simulink model "3_Pose_integration_R_L"  (R2020b)
settings: Solver=FixedStepDiscrete  StartTime=0.0  StopTime=60  FixedStep=0.02  RelTol=1e-3  EnableMultiTasking=on
InitFcn:
  | load('Encoder_Data.mat')
StopFcn:
  | I = imread('Enviroment.png');
  | x = [0 35.9];
  | y=[23.31 0];
  | image(I,'XData',x,'YData',y);
  | axis xy;
  | hold on
  | plot (X.Data, Y.Data,'b');
  | plot (X1.Data, Y1.Data,'r');
undefined symbols (not defined in the file or in its folder): DiscIntNeverNeededParam, Ts
libraries: simulink x3
settings Model: Creator=antonio  LastModifiedBy=antonio
settings DataIOCC: LimitDataPoints=on  SaveFormat=Array  ReturnWorkspaceOutputs=off
settings OptimizationCC: LifeSpan=inf
settings DebuggingCC: UnderspecifiedInitializationDetection=Classic  MergeDetectMultiDrivingBlocksExec=none  SolverPrmCheckMsg=warning  StateNameClashWarn=warning  SFUnexpectedBacktrackingDiag=warning  SFNoUnconditionalDefaultTransitionDiag=warning  SFExecutionAtInitializationDiag=none  ArithmeticOperatorsInVariantConditions=warning
settings HardwareCC: ProdBitPerPointer=32  ProdBitPerSizeT=32  ProdBitPerPtrDiffT=32  ProdLargestAtomicFloat=None  ProdIntDivRoundTo=Undefined  ProdEndianess=Unspecified  ProdWordSize=32  ProdHWDeviceType=32-bit Generic
settings ModelReferenceCC: PropagateSignalLabelsOutOfModel=off
settings SFSimCC: SimUseLocalCustomCode=off  CustomCodeUndefinedFunction=UseInterfaceOnly
settings RTWCC: RTWUseLocalCustomCode=off
settings CodeAppCC: StateflowObjectComments=on
settings GRTTargetCC: TargetLangStandard=C89/C90 (ANSI)
settings ConfigComp: CovMetricSettings=dw  CovSaveCumulativeToWorkspaceVar=on  CovSaveSingleToWorkspaceVar=on  CovExternalEMLEnable=off

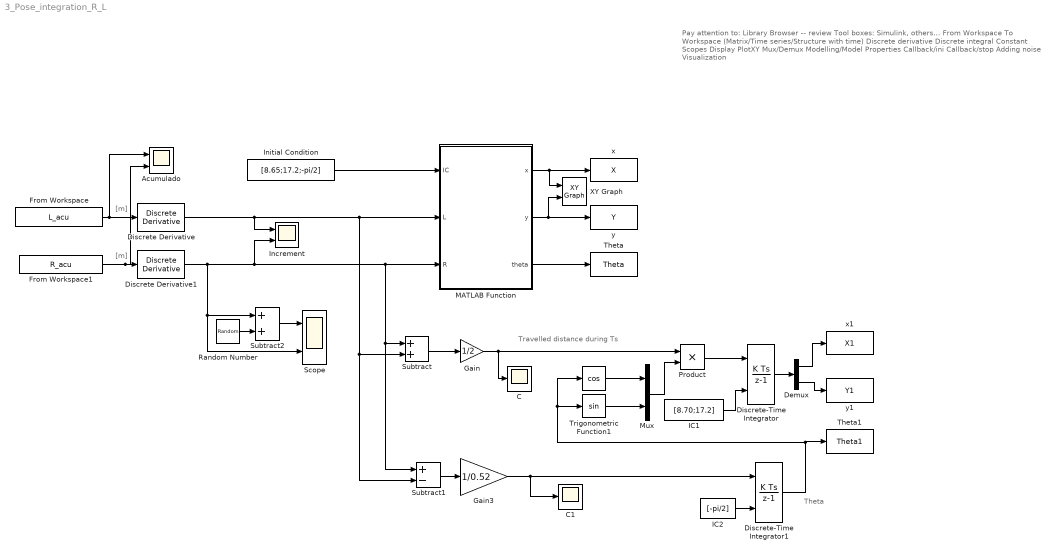
== system 3_Pose_integration_R_L ==
  note: Theta
  note: Pay attention to:
      |
      | Library Browser -- review
      | Tool boxes: Simulink, others...
      | From Workspace
      | To Workspace (Matrix/Time series/Structure with time)
      | Discrete derivative
      | Discrete integral
      | Constant
      | Scopes
      | Display
      | PlotXY
      | Mux/Demux
      | Modelling/Model Properties
      | Callback/ini
      | Callback/stop
      | Adding noise
      | Visualization
  note: Travelled distance during Ts
  note: [m]
  note: [m]
  " " : Trigonometry  Operator=cos
  Acumulado : Scope  NumInputPorts=2
  C : Scope
  C1 : Scope
  Demux : Demux  Outputs=2
  Discrete Derivative : simulink/Discrete/Discrete Derivative  gainval=Ts  ICPrevScaledInput=0.0  OutMin=[]  OutMax=[]  OutDataType=fixdt(1, 16)  OutScaling=2^-10  DoSatur=off
  Discrete Derivative1 : simulink/Discrete/Discrete Derivative  gainval=Ts  ICPrevScaledInput=0.0  OutMin=[]  OutMax=[]  OutDataType=fixdt(1, 16)  OutScaling=2^-10  DoSatur=off
  Discrete-Time Integrator : DiscreteIntegrator  gainval=1/Ts  InitialConditionSource=external  SampleTime=Ts  ICPrevOutput=DiscIntNeverNeededParam  ICPrevScaledInput=DiscIntNeverNeededParam
  Discrete-Time Integrator1 : DiscreteIntegrator  gainval=1/Ts  InitialConditionSource=external  SampleTime=Ts  ICPrevOutput=DiscIntNeverNeededParam  ICPrevScaledInput=DiscIntNeverNeededParam
  From Workspace : FromWorkspace  VariableName=L_acu  SampleTime=Ts
  From Workspace1 : FromWorkspace  VariableName=R_acu  SampleTime=Ts
  Gain : Gain  Gain=1/2
  Gain3 : Gain  Gain=1/0.52
  IC1 : Constant  Value=[8.70;17.2]
  IC2 : Constant  Value=[-pi/2]
  Increment : Scope  NumInputPorts=2
  Initial Condition : Constant  Value=[8.65;17.2;-pi/2]
  MATLAB Function : MATLAB Function  TreatAsAtomicUnit=on
  Mux : Mux  Inputs=2
  Product : Product
  Random Number : RandomNumber  Variance=0.005^2  SampleTime=Ts
  Scope : Scope  NumInputPorts=2
  Subtract : Sum
  Subtract1 : Sum  Inputs=+-
  Subtract2 : Sum
  Theta : ToWorkspace  VariableName=Theta  SaveFormat=Timeseries  SampleTime=-1
  Theta1 : ToWorkspace  VariableName=Theta1  SaveFormat=Timeseries  SampleTime=-1
  Trigonometric Function1 : Trigonometry
  XY Graph : simulink/Sinks/XY Graph  xmin=5  xmax=25  ymin=2  ymax=18  st=-1
  x : ToWorkspace  VariableName=X  SaveFormat=Timeseries  SampleTime=-1
  x1 : ToWorkspace  VariableName=X1  SaveFormat=Timeseries  SampleTime=-1
  y : ToWorkspace  VariableName=Y  SaveFormat=Timeseries  SampleTime=-1
  y1 : ToWorkspace  VariableName=Y1  SaveFormat=Timeseries  SampleTime=-1
  wires:
  Initial Condition/1 -> MATLAB Function/1(IC)
  MATLAB Function/3(theta) -> Theta/1
  MATLAB Function/2(y) -> XY Graph/2, y/1
  MATLAB Function/1(x) -> XY Graph/1, x/1
  From Workspace1/1 -> Acumulado/2, Discrete Derivative1/1
  From Workspace/1 -> Acumulado/1, Discrete Derivative/1
  Subtract/1 -> Gain/1
  Gain/1 -> C/1, Product/1
  Trigonometric Function1/1 -> Mux/2
  " "/1 -> Mux/1
  Mux/1 -> Product/2
  Subtract1/1 -> Gain3/1
  Product/1 -> Discrete-Time Integrator/1
  IC1/1 -> Discrete-Time Integrator/2
  Discrete-Time Integrator/1 -> Demux/1
  Demux/1 -> x1/1
  Demux/2 -> y1/1
  Discrete-Time Integrator1/1 -> " "/1, Trigonometric Function1/1, Theta1/1
  Gain3/1 -> C1/1, Discrete-Time Integrator1/1
  IC2/1 -> Discrete-Time Integrator1/2
  Discrete Derivative/1 -> Increment/1, MATLAB Function/2(L), Subtract1/2, Subtract/2
  Discrete Derivative1/1 -> Scope/2, Subtract2/1, Increment/2, Subtract1/1, Subtract/1, MATLAB Function/3(R)
  Random Number/1 -> Subtract2/2
  Subtract2/1 -> Scope/1

== matlab function 3_Pose_integration_R_L/MATLAB Function ==
  data: x output; y output; theta output; IC input; L input; R input
function [x,y,theta] = fcn(IC,L,R) 
% IC->Initial Condition [xo,yo,th0]
% R and L are the incremental displacements of wheels [m]
persistent x_w y_w suma_theta %  internal variable to be mantain its values

ts=0.02; % sample time
W=0.52%2S

%%%%%%%%%%%%%%%%%%%%%%%%%%%%%%%%%%%%%%%%%%%%%%%%%%%%%%%%%%%%%%%%%%%%%%%%%%
% %%%%%%%%%%%%%%   Read Initial condition   %%%%%%%%%%%%%%%%%%%%%%%%%%%%%%
x_ini=IC(1);
y_ini=IC(2);
theta_ini=IC(3);
%%%%%%%%%%%%%%%%%%%%%%%%%%%%%%%%%%%%%%%%%%%%%%%%%%%%%%%%%%%%%%%%%%%%%%%%%%
%%%%%%%%%%%%%%%   variable initialitation  %%%%%%%%%%%%%%%%%%%%%%%%%%%%%%
if isempty (x_w)
    x_w=x_ini;
end
if isempty (y_w)
    y_w=y_ini;
end
if isempty (suma_theta)
    suma_theta=theta_ini;
end
%%%%%%%%%%%%%%%%%%%%%%%%%%%%%%%%%%%%%%%%%%%%%%%%%%%%%%%%%%%%%%%%%%%%%%%%%%
%%%%%%%%%%%%%%%%%  compute the odometry    %%%%%%%%%%%%%%%%%%%%%%%%%%%%%%%
delta_th=(R-L)/W;
delta_d=(R+L)/2;
%%%%%%%%%%%%%%%%%%%%%%%%%%%%%%%%%%%%%%%%%%%%%%%%%%%%%%%%%%%%%%%%%%%%%%%%%%
%%%%%%%%%%%%%%%%%  integration of the robot pose %%%%%%%%%%%%%%%%%%%%%%%%%%
x_w=x_w + delta_d*cos(suma_theta)
y_w=y_w + delta_d*sin(suma_theta)
suma_theta=mod(suma_theta+delta_th,2*pi); 
%%%%%%%%%%%%%%%%%%%%%%%%%%%%%%%%%%%%%%%%%%%%%%%%%%%%%%%%%%%%%%%%%%%%%%%%%%
%%%%%%%%%%%%%%%%%  output variable %%%%%%%%%%%%%%%%%%%%%%%%%%%%%%%%%%%%%%%

x=x_w;
y=y_w;
theta=suma_theta

end
